simulink model "sla_vip_filter_enb"  (R2015b)
settings: Solver=FixedStepDiscrete  StartTime=0.0  StopTime=1  RelTol=1e-3
PreLoadFcn:
  | Param_vip_pixel1
values from neighbouring files (symbols this model uses):
  Hr = fspecial('unsharp')    [Param_vip_pixel1.m]
libraries: visionsinks x5, dspsigattribs x3, visionutilities x2, dspvision x1, visionfilter x1
settings Model: Creator=amatsumo  LastModifiedBy=amatsumo
settings DataIOCC: SaveFormat=Array  SignalLoggingSaveFormat=ModelDataLogs
settings OptimizationCC: BlockReduction=off  ConditionallyExecuteInputs=off  ExpressionDepthLimit=2147483647
settings DebuggingCC: UnderspecifiedInitializationDetection=Classic  MergeDetectMultiDrivingBlocksExec=none  SolverPrmCheckMsg=warning  FcnCallInpInsideContextMsg=UseLocalSettings  StateNameClashWarn=warning
settings HardwareCC: ProdBitPerPointer=32  ProdLargestAtomicFloat=None  ProdIntDivRoundTo=Undefined  ProdEndianess=Unspecified  ProdWordSize=32  ProdHWDeviceType=ASIC/FPGA->ASIC/FPGA  TargetBitPerPointer=64  TargetLongLongMode=on  TargetIntDivRoundTo=Zero  TargetEndianess=LittleEndian  TargetWordSize=64  TargetHWDeviceType=MATLAB Host  ProdEqTarget=off
settings GRTTargetCC: GeneratePreprocessorConditionals=Disable all  CombineOutputUpdateFcns=off  GRTInterface=on
settings ConfigComp: CovModelRefEnable=Off  CovSFcnEnable=off

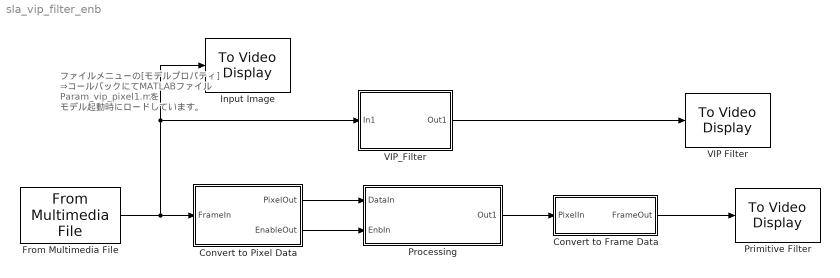
== system sla_vip_filter_enb ==
  note: ファイルメニューの[モデルプロパティ]
      | ⇒コールバックにてMATLABファイル
      | Param_vip_pixel1.mを
      | モデル起動時にロードしています。
  Convert to Frame Data : Subsystem
  Convert to Pixel Data : Subsystem
  From Multimedia File : dspvision/From Multimedia File  inputFilename=vipmen.avi  loop=on  numPlays=inf  outputStreams=Video only  videoDataType=uint8  audioDataType=int16  inheritSampleTime=off  userDefinedSampleTime=1/24  noAudioOutput=off  isIntensityVideo=off  fourcc=Intensity  colorVideoFormat=One multidimensional signal  outputEOF=off  dataOrg=Column-major  audioFrameSize=1024  computeAudioFrameSize=off  outSamplingMode=Frame based
  Input Image : visionsinks/To Video Display  windowSizeMode=True size (1:1)  openAtMdlStart=on  fullScreen=off  videoWindowX=367  videoWindowY=50  saveWindowSize=off  videoWindowWidth=160  videoWindowHeight=120  inputColorFormat=RGB  inputType=Obsolete  imagePorts=One multidimensional signal  OutputDevice=On-screen video monitor  dataOrg=Column-major  isWindowOpen=on
  Primitive Filter : visionsinks/To Video Display  windowSizeMode=True size (1:1)  openAtMdlStart=on  fullScreen=off  videoWindowX=920  videoWindowY=48  saveWindowSize=off  videoWindowWidth=180  videoWindowHeight=130  inputColorFormat=RGB  inputType=Obsolete  imagePorts=One multidimensional signal  OutputDevice=On-screen video monitor  dataOrg=Column-major  isWindowOpen=on
  Processing : Subsystem
  VIP Filter : visionsinks/To Video Display  windowSizeMode=True size (1:1)  openAtMdlStart=on  fullScreen=off  videoWindowX=642  videoWindowY=48  saveWindowSize=off  videoWindowWidth=160  videoWindowHeight=120  inputColorFormat=RGB  inputType=Obsolete  imagePorts=One multidimensional signal  OutputDevice=On-screen video monitor  dataOrg=Column-major  isWindowOpen=on
  VIP_Filter : Subsystem
  wires:
  From Multimedia File/1 -> Convert to Pixel Data/1(FrameIn), VIP_Filter/1(In1), Input Image/1
  VIP_Filter/1(Out1) -> VIP Filter/1
  Convert to Frame Data/1(FrameOut) -> Primitive Filter/1
  Convert to Pixel Data/1(PixelOut) -> Processing/1(DataIn)
  Processing/1(Out1) -> Convert to Frame Data/1(PixelIn)
  Convert to Pixel Data/2(EnableOut) -> Processing/2(EnbIn)

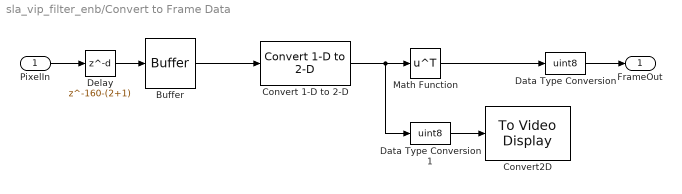
== system sla_vip_filter_enb/Convert to Frame Data ==
  PixelIn : Inport
  Buffer : Buffer  N=180*130  TreatMby1Signals=One channel
  Convert 1-D to 2-D : dspsigattribs/Convert 1-D to 2-D  M=180  N=130  frameBasedOut=off
  Convert2D : visionsinks/To Video Display  windowSizeMode=True size (1:1)  openAtMdlStart=on  fullScreen=off  videoWindowX=807  videoWindowY=275  saveWindowSize=off  videoWindowWidth=130  videoWindowHeight=180  inputColorFormat=RGB  inputType=Obsolete  imagePorts=One multidimensional signal  OutputDevice=On-screen video monitor  dataOrg=Column-major  isWindowOpen=on
  Data Type Conversion : DataTypeConversion  OutDataTypeStr=uint8  SaturateOnIntegerOverflow=on
  Data Type Conversion1 : DataTypeConversion  OutDataTypeStr=uint8  SaturateOnIntegerOverflow=on
  Delay : Delay  DelayLength=160-(2+1)  InitialCondition=0
  Math Function : Math  Operator=transpose  SaturateOnIntegerOverflow=on
  FrameOut : Outport
  wires:
  Data Type Conversion/1 -> FrameOut/1
  Delay/1 -> Buffer/1
  Math Function/1 -> Data Type Conversion/1
  PixelIn/1 -> Delay/1
  Convert 1-D to 2-D/1 -> Math Function/1, Data Type Conversion1/1
  Buffer/1 -> Convert 1-D to 2-D/1
  Data Type Conversion1/1 -> Convert2D/1

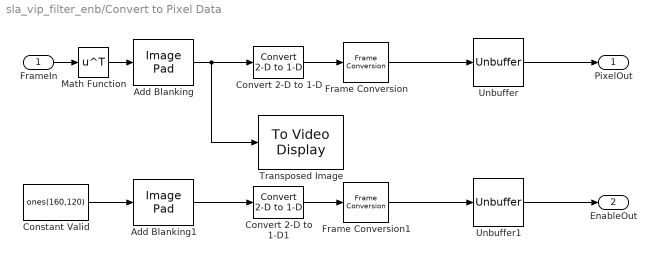
== system sla_vip_filter_enb/Convert to Pixel Data ==
  FrameIn : Inport
  Add Blanking : visionutilities/Image Pad  method=Constant  valSrc=Specify via dialog  value=0  spec=Pad size  rowDirection=Both left and right  outRowsMode=User-specified  rowSize=[0 10]  outColSize=10  colDirection=Both top and bottom  outColsMode=User-specified  colSize=[0 20]  outRowSize=12  trunc_flag=None
  Add Blanking1 : visionutilities/Image Pad  method=Constant  valSrc=Specify via dialog  value=0  spec=Pad size  rowDirection=Both left and right  outRowsMode=User-specified  rowSize=[0 10]  outColSize=10  colDirection=Both top and bottom  outColsMode=User-specified  colSize=[0 20]  outRowSize=12  trunc_flag=None
  Constant Valid : Constant  Value=ones(160,120)  OutDataTypeStr=boolean  SampleTime=1/24
  Convert 2-D to 1-D : dspsigattribs/Convert 2-D to 1-D
  Convert 2-D to 1-D1 : dspsigattribs/Convert 2-D to 1-D
  Frame Conversion : FrameConversion  InheritSamplingMode=off
  Frame Conversion1 : FrameConversion  InheritSamplingMode=off
  Math Function : Math  Operator=transpose  SaturateOnIntegerOverflow=on
  Transposed Image : visionsinks/To Video Display  windowSizeMode=True size (1:1)  openAtMdlStart=on  fullScreen=off  videoWindowX=582  videoWindowY=275  saveWindowSize=off  videoWindowWidth=130  videoWindowHeight=180  inputColorFormat=RGB  inputType=Obsolete  imagePorts=One multidimensional signal  OutputDevice=On-screen video monitor  dataOrg=Column-major  isWindowOpen=on
  Unbuffer : Unbuffer  SampleBasedProcessing=Same as frame based
  Unbuffer1 : Unbuffer  SampleBasedProcessing=Same as frame based
  PixelOut : Outport
  EnableOut : Outport  Port=2
  wires:
  Math Function/1 -> Add Blanking/1
  Unbuffer/1 -> PixelOut/1
  FrameIn/1 -> Math Function/1
  Convert 2-D to 1-D/1 -> Frame Conversion/1
  Frame Conversion/1 -> Unbuffer/1
  Add Blanking/1 -> Convert 2-D to 1-D/1, Transposed Image/1
  Constant Valid/1 -> Add Blanking1/1
  Convert 2-D to 1-D1/1 -> Frame Conversion1/1
  Frame Conversion1/1 -> Unbuffer1/1
  Add Blanking1/1 -> Convert 2-D to 1-D1/1
  Unbuffer1/1 -> EnableOut/1

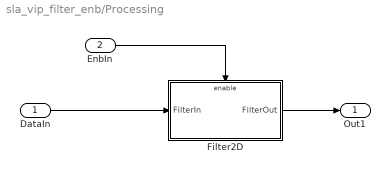
== system sla_vip_filter_enb/Processing ==
  DataIn : Inport
  EnbIn : Inport  Port=2
  Filter2D : Subsystem
  Out1 : Outport
  wires:
  DataIn/1 -> Filter2D/1(FilterIn)
  Filter2D/1(FilterOut) -> Out1/1
  EnbIn/1 -> Filter2D/Enable

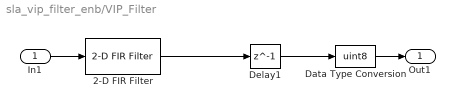
== system sla_vip_filter_enb/VIP_Filter ==
  In1 : Inport
  2-D FIR Filter : visionfilter/2-D FIR Filter  separable=off  filtSrc=Specify via dialog  filterMtrx=Hr  verticalFilter=[4 0]  horizontalFilter=[4 0]  outSize=Same as input port I  padType=Constant  padSrc=Specify via dialog  padVal=0  method=Convolution  firstCoeffMode=Binary point scaling  firstCoeffWordLength=7  firstCoeffFracLength=3  firstCoeffSignedness=Signed  firstCoeffDataTypeStr=fixdt(1,7,3)  firstCoeffLastDataTypeStr=fixdt(1,7,3)  firstCoeffMin=[]  firstCoeffMax=[]  outputMode=Binary point scaling  outputWordLength=19  outputFracLength=8  outputSignedness=Auto  outputDataTypeStr=fixdt([],19,8)  outputLastDataTypeStr=fixdt([],19,8)  outputMin=[]  outputMax=[]  accumDataTypeStr=Inherit: Same as product output  accumLastDataTypeStr=Inherit: Same as product output  prodOutputMode=Binary point scaling  prodOutputWordLength=15  prodOutputFracLength=3  prodOutputDataTypeStr=fixdt([],15,3)  prodOutputLastDataTypeStr=fixdt([],15,3)  roundingMode=Floor  overflowMode=on
  Data Type Conversion : DataTypeConversion  OutDataTypeStr=uint8  SaturateOnIntegerOverflow=on
  Delay1 : Delay  DelayLength=1  InitialCondition=0  UseCircularBuffer=on
  Out1 : Outport
  wires:
  Delay1/1 -> Data Type Conversion/1
  2-D FIR Filter/1 -> Delay1/1
  In1/1 -> 2-D FIR Filter/1
  Data Type Conversion/1 -> Out1/1

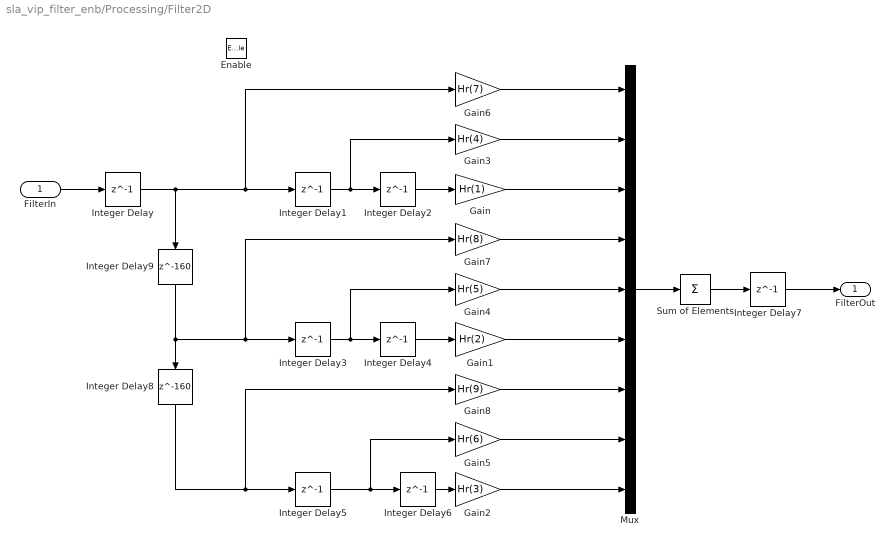
== system sla_vip_filter_enb/Processing/Filter2D ==
  FilterIn : Inport
  Enable : EnablePort
  Gain : Gain  Gain=Hr(1)  ParamDataTypeStr=fixdt(1,7,3)
  Gain1 : Gain  Gain=Hr(2)  ParamDataTypeStr=fixdt(1,7,3)
  Gain2 : Gain  Gain=Hr(3)  ParamDataTypeStr=fixdt(1,7,3)
  Gain3 : Gain  Gain=Hr(4)  ParamDataTypeStr=fixdt(1,7,3)  RndMeth=Nearest
  Gain4 : Gain  Gain=Hr(5)  ParamDataTypeStr=fixdt(1,7,3)
  Gain5 : Gain  Gain=Hr(6)  ParamDataTypeStr=fixdt(1,7,3)
  Gain6 : Gain  Gain=Hr(7)  ParamDataTypeStr=fixdt(1,7,3)
  Gain7 : Gain  Gain=Hr(8)  ParamDataTypeStr=fixdt(1,7,3)
  Gain8 : Gain  Gain=Hr(9)  ParamDataTypeStr=fixdt(1,7,3)
  Integer Delay{,1..7} (8 alike) : Delay  DelayLength=1  InputProcessing=Inherited
  Integer Delay8 : Delay  DelayLength=160  InputProcessing=Inherited
  Integer Delay9 : Delay  DelayLength=160  InputProcessing=Inherited
  Mux : Mux  Inputs=9
  Sum of Elements : Sum  Inputs=+  RndMeth=Nearest
  FilterOut : Outport  InitialOutput=0
  wires:
  Sum of Elements/1 -> Integer Delay7/1
  Mux/1 -> Sum of Elements/1
  Integer Delay3/1 -> Gain4/1, Integer Delay4/1
  Integer Delay5/1 -> Gain5/1, Integer Delay6/1
  Integer Delay8/1 -> Gain8/1, Integer Delay5/1
  Integer Delay9/1 -> Gain7/1, Integer Delay3/1, Integer Delay8/1
  Integer Delay1/1 -> Gain3/1, Integer Delay2/1
  FilterIn/1 -> Integer Delay/1
  Gain6/1 -> Mux/1
  Integer Delay/1 -> Gain6/1, Integer Delay1/1, Integer Delay9/1
  Integer Delay7/1 -> FilterOut/1
  Integer Delay2/1 -> Gain/1
  Gain3/1 -> Mux/2
  Gain/1 -> Mux/3
  Gain7/1 -> Mux/4
  Gain4/1 -> Mux/5
  Integer Delay4/1 -> Gain1/1
  Gain1/1 -> Mux/6
  Integer Delay6/1 -> Gain2/1
  Gain2/1 -> Mux/9
  Gain8/1 -> Mux/7
  Gain5/1 -> Mux/8
